simulink model "deadbeat"  (R2018b)
settings: Solver=ode1  StartTime=0.0  StopTime=1  FixedStep=1e-6  RelTol=1e-4
undefined symbols (not defined in the file): Ba, DiscIntNeverNeededParam, flux, Ki, Kp, Ld, Lq, R, Ts
libraries: powerlib x4, simulink x1
settings Model: SimulationMode=accelerator  ExtModeTrigMode=oneshot  ExtModeArmWhenConnect=off  ExtModeAutoUpdateStatusClock=off  Creator=Administrador  LastModifiedBy=123
settings DataIOCC: SaveFormat=Array  SignalLoggingSaveFormat=ModelDataLogs  SignalLoggingName=sigsOut
settings OptimizationCC: BlockReduction=off  BooleanDataType=off  ExpressionDepthLimit=2147483647  InitFltsAndDblsToZero=on  LifeSpan=inf
settings DebuggingCC: SaveWithParameterizedLinksMsg=none  UnderspecifiedInitializationDetection=Classic  MergeDetectMultiDrivingBlocksExec=none  SignalResolutionControl=TryResolveAllWithWarning  MultiTaskDSMMsg=warning  MultiTaskCondExecSysMsg=none  FcnCallInpInsideContextMsg=warning  StateNameClashWarn=warning  LibraryContextMissingDiagnostic=none  SFUnexpectedBacktrackingDiag=warning  SFNoUnconditionalDefaultTransitionDiag=warning  SFExecutionAtInitializationDiag=none
settings HardwareCC: ProdBitPerPointer=32  ProdBitPerSizeT=32  ProdBitPerPtrDiffT=32  ProdLargestAtomicFloat=None  ProdIntDivRoundTo=Undefined  ProdEndianess=Unspecified  ProdWordSize=32  ProdHWDeviceType=32-bit Generic  TargetUnknown=on
settings ModelReferenceCC: PropagateSignalLabelsOutOfModel=off
settings SFSimCC: SimUseLocalCustomCode=off
settings RTWCC: RTWUseLocalCustomCode=off
settings CodeAppCC: StateflowObjectComments=on
settings GRTTargetCC: TargetFcnLib=ansi_tfl_tmw.mat  TargetLangStandard=C89/C90 (ANSI)  GeneratePreprocessorConditionals=Disable all  CombineOutputUpdateFcns=off  GRTInterface=on
settings ConfigComp: CovMetricSettings=dw  CovHtmlReporting=on  CovSaveCumulativeToWorkspaceVar=on  CovSaveSingleToWorkspaceVar=on  CovExternalEMLEnable=off  CovSFcnEnable=off

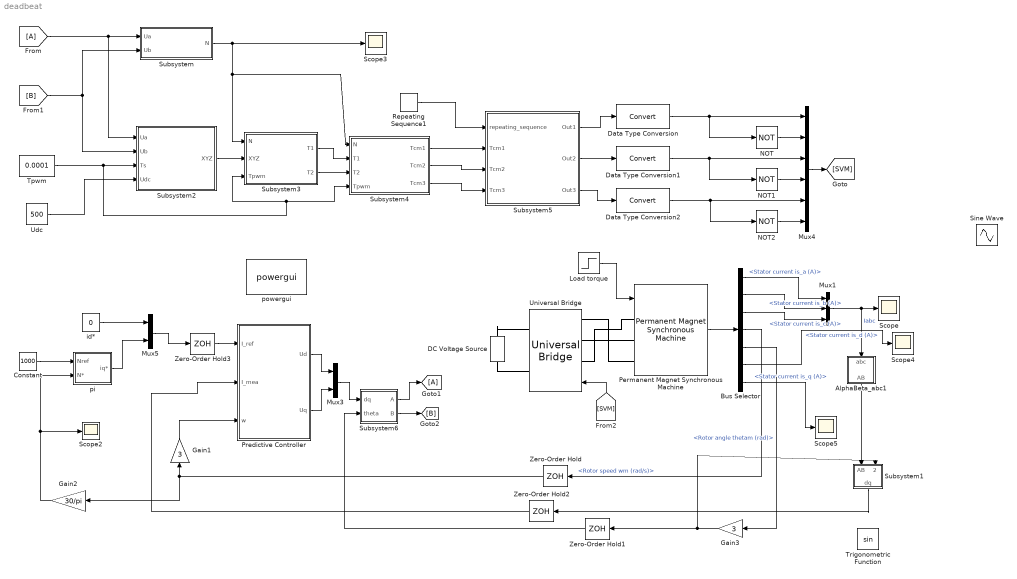
== system deadbeat ==
  AlphaBeta_abc1 : Subsystem
  Bus Selector : BusSelector  OutputSignals=Stator current is_a (A),Stator current is_b (A),Stator current is_c (A),Rotor speed wm (rad/s),Rotor angle thetam (rad),Stator current is_d (A),Stator current is_q (A)
  Constant : Constant  Value=1000
  DC Voltage Source : powerlib/Electrical Sources/DC Voltage Source  Amplitude=500  Measurements=None
      settings: SourceProductName=Simscape Electrical
  Data Type Conversion : DataTypeConversion
  Data Type Conversion1 : DataTypeConversion
  Data Type Conversion2 : DataTypeConversion
  Gain1 : Gain  Gain=3
  Gain2 : Gain  Gain=30/pi
  Gain3 : Gain  Gain=3
  Load torque : Step  Time=0.35  After=5  SampleTime=5e-6
  Mux1 : Mux  Inputs=3
  Mux3 : Mux  Inputs=2
  Mux4 : Mux  Inputs=6
  Mux5 : Mux  Inputs=2
  NOT : Logic  Operator=NOT  IconShape=distinctive  AllPortsSameDT=off  OutDataTypeStr=boolean
  NOT1 : Logic  Operator=NOT  IconShape=distinctive  AllPortsSameDT=off  OutDataTypeStr=boolean
  NOT2 : Logic  Operator=NOT  IconShape=distinctive  AllPortsSameDT=off  OutDataTypeStr=boolean
  Permanent Magnet Synchronous Machine : powerlib/Machines/Permanent Magnet Synchronous Machine  NbPhases=3  FluxDistribution=Sinusoidal  RotorType=Salient-pole  MechanicalLoad=Torque Tm  PresetModel=No  ShowDetailedParameters=on  MeasurementBus=off  Resistance=1.4  Inductance=8.5e-3  dqInductances=[4e-3,6e-3]  La=0.006  MachineConstant=Flux linkage established by magnets (V.s)  Flux=0.09356  VoltageCst=50.9097  TorqueCst=0.42102  Flat=120  Mechanical=[0.0004 0.008 3 0]  PolePairs=4  InitialConditions=[0,0, 0,0]  InitialConditions5ph=[0 0 0 0 0 0]  TsPowergui=0  TsBlock=-1  RefAngle=Aligned with phase A axis (original Park)
  Predictive Controller : MATLAB Function  TreatAsAtomicUnit=on  SystemSampleTime=5e-6
  Repeating Sequence1 : simulink/Sources/Repeating Sequence  rep_seq_t=[0 5e-5 1e-4]  rep_seq_y=[0 5e-5 0]
  Scope{,2..5} (5 alike) : Scope
  Sine Wave : Sin  TimeSource=Use external signal  SampleTime=0
  Subsystem : Subsystem
  Subsystem1 : Subsystem
  Subsystem2 : Subsystem
  Subsystem3 : Subsystem
  Subsystem4 : Subsystem
  Subsystem5 : Subsystem
  Subsystem6 : Subsystem
  Tpwm : Constant  Value=0.0001
  Trigonometric Function : Trigonometry
  "Udc " : Constant  Value=500
  Universal Bridge : powerlib/Power Electronics/Universal Bridge  Arms=3  SnubberResistance=1e5  SnubberCapacitance=inf  Device=IGBT / Diodes  Ron=1e-3  Lon=0  ForwardVoltages="[  0  0  ]"  ForwardVoltage=0  GTOparameters=[ 10e-6 , 20e-6 ]  IGBTparameters=[ 1e-6 , 2e-6 ]  Measurements=None  Measurements_2=None  converterType=Rectifier
      settings: SourceProductName=Simscape Electrical
  Zero-Order Hold{,1..3} (4 alike) : ZeroOrderHold  SampleTime=5e-6
  id* : Constant  Value=0
  pi : Subsystem
  powergui : powerlib/powergui  Priority=1  SimulationMode=Discrete  SampleTime=1e-6  frequency=60  Iterations=50  frequencyindice=0  Pbase=100e6  ErrMax=1e-4  UnitsV=kV  UnitsW=MW  buscounter=0  FunctionMessages=off  echomessages=off  EnableUseOfTLC=off  CurrentSourceSwitches=off  DisableSnubberDevices=off  DisableRonSwitches=off  DisableVfSwitches=off  DisplayEquations=off  SolverType=Tustin  Interpol=off  ExternalGateDelay=off  methode=off  Ts=0  x0status=blocks  SPID=off  SwTol=0  HookPort=off  RestoreLinks=warning  ResistiveCurrentMeasurement=off  Frange=[0:2:500]  Ylog=off  Xlog=on  ShowGrid=off  save=off  variable=ZData  structure=ScopeData1  ZoomFFT=off  StartTime=0.05  cycles=1  DisplayStyle=1  fundamental=50  FreqAxis=off  MaxFrequency=2000  frequencyindicesteady=1  RmsSteady=1  display=off
  wires:
  Mux1/1 -> Scope/1, AlphaBeta_abc1/1(abc)  "Iabc"
  Permanent Magnet Synchronous Machine/1 -> Bus Selector/1
  Bus Selector/1 -> Mux1/1  "<Stator current is_a (A)>"
  Bus Selector/2 -> Mux1/2  "<Stator current is_b (A)>"
  Bus Selector/3 -> Mux1/3  "<Stator current is_c (A)>"
  Constant/1 -> pi/1(Nref)
  Gain2/1 -> pi/2(N*), Scope2/1
  Bus Selector/4 -> Zero-Order Hold/1  "<Rotor speed wm (rad/s)>"
  id*/1 -> Mux5/1
  pi/1(iq*) -> Mux5/2
  Mux5/1 -> Zero-Order Hold3/1
  Gain1/1 -> Predictive Controller/3(w)
  Bus Selector/5 -> Gain3/1  "<Rotor angle thetam (rad)>"
  Gain3/1 -> Zero-Order Hold1/1, Subsystem1/2(theta)
  AlphaBeta_abc1/1(AB) -> Subsystem1/1(AB)
  Subsystem1/1(dq) -> Zero-Order Hold2/1
  Subsystem4/1(Tcm1) -> Subsystem5/2(Tcm1)
  Subsystem/1(N) -> Subsystem4/1(N), Subsystem3/1(N), Scope3/1
  Data Type Conversion/1 -> NOT/1, Mux4/1
  Mux4/1 -> [SVM]
  Subsystem3/2("T2 ") -> Subsystem4/3(T2)
  Subsystem4/2(Tcm2) -> Subsystem5/3(Tcm2)
  NOT2/1 -> Mux4/6
  Subsystem5/2(Out2) -> Data Type Conversion1/1
  Data Type Conversion2/1 -> NOT2/1, Mux4/5
  Subsystem5/3(Out3) -> Data Type Conversion2/1
  NOT/1 -> Mux4/2
  Repeating Sequence1/1 -> Subsystem5/1(repeating_sequence)
  Tpwm/1 -> Subsystem4/4(Tpwm), Subsystem3/3(Tpwm), Subsystem2/3(Ts)
  Subsystem2/1(XYZ) -> Subsystem3/2(XYZ)
  "Udc "/1 -> Subsystem2/4(Udc)
  Data Type Conversion1/1 -> NOT1/1, Mux4/3
  Subsystem5/1(Out1) -> Data Type Conversion/1
  [B] -> Subsystem2/2(Ub), Subsystem/2(Ub)
  NOT1/1 -> Mux4/4
  [A] -> Subsystem2/1(Ua), Subsystem/1(Ua)
  Subsystem3/1(T1) -> Subsystem4/2(T1)
  Subsystem4/3(Tcm3) -> Subsystem5/4(Tcm3)
  [SVM] -> Universal Bridge/1
  Predictive Controller/1(Ud) -> Mux3/1
  Predictive Controller/2(Uq) -> Mux3/2
  Mux3/1 -> Subsystem6/1(dq)
  Subsystem6/2(B) -> [B]
  Subsystem6/1(A) -> [A]
  Zero-Order Hold/1 -> Gain2/1, Gain1/1
  Zero-Order Hold1/1 -> Subsystem6/2(theta)
  Zero-Order Hold2/1 -> Predictive Controller/2(I_mea)
  Zero-Order Hold3/1 -> Predictive Controller/1(I_ref)
  Bus Selector/6 -> Scope4/1  "<Stator current is_d (A)>"
  Bus Selector/7 -> Scope5/1  "<Stator current is_q (A)>"
  Load torque/1 -> Permanent Magnet Synchronous Machine/1
  connections:
  DC Voltage Source/RConn1 -- Universal Bridge/RConn1
  DC Voltage Source/LConn1 -- Universal Bridge/RConn2
  Universal Bridge/LConn3 -- Permanent Magnet Synchronous Machine/LConn3
  Permanent Magnet Synchronous Machine/LConn2 -- Universal Bridge/LConn2
  Universal Bridge/LConn1 -- Permanent Magnet Synchronous Machine/LConn1

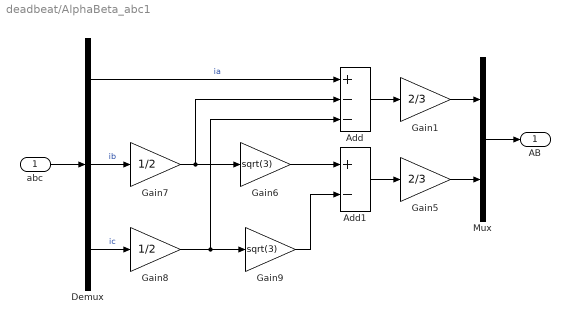
== system deadbeat/AlphaBeta_abc1 ==
  abc : Inport
  Add : Sum  Inputs=+--
  Add1 : Sum  Inputs=+-
  Demux : Demux  Outputs=3
  Gain1 : Gain  Gain=2/3
  Gain5 : Gain  Gain=2/3
  Gain6 : Gain  Gain=sqrt(3)
  Gain7 : Gain  Gain=1/2
  Gain8 : Gain  Gain=1/2
  Gain9 : Gain  Gain=sqrt(3)
  Mux : Mux  Inputs=2
  AB : Outport
  wires:
  abc/1 -> Demux/1
  Demux/2 -> Gain7/1  "ib"
  Demux/3 -> Gain8/1  "ic"
  Add/1 -> Gain1/1
  Gain7/1 -> Gain6/1, Add/2
  Gain8/1 -> Gain9/1, Add/3
  Gain6/1 -> Add1/1
  Gain9/1 -> Add1/2
  Demux/1 -> Add/1  "ia"
  Add1/1 -> Gain5/1
  Gain1/1 -> Mux/1
  Gain5/1 -> Mux/2
  Mux/1 -> AB/1

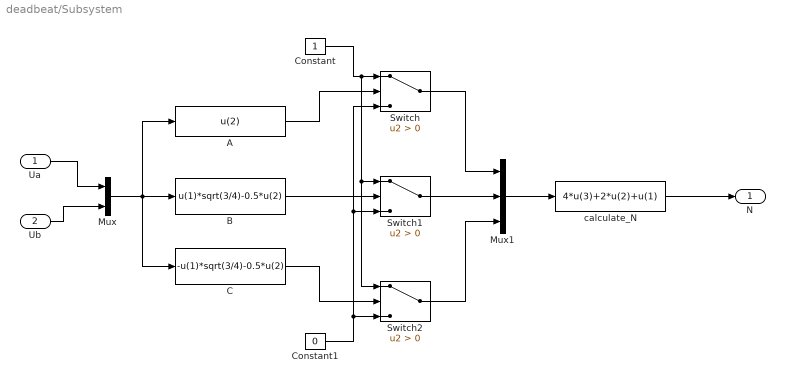
== system deadbeat/Subsystem ==
  Ua : Inport
  Ub : Inport  Port=2
  A : Fcn  Expr=u(2)
  B : Fcn  Expr=u(1)*sqrt(3/4)-0.5*u(2)
  C : Fcn  Expr=-u(1)*sqrt(3/4)-0.5*u(2)
  Constant : Constant
  Constant1 : Constant  Value=0
  Mux : Mux  Inputs=2
  Mux1 : Mux  Inputs=3
  Switch : Switch  Criteria=u2 > Threshold
  Switch1 : Switch  Criteria=u2 > Threshold
  Switch2 : Switch  Criteria=u2 > Threshold
  calculate_N : Fcn  Expr=4*u(3)+2*u(2)+u(1)
  N : Outport
  wires:
  Ua/1 -> Mux/1
  Ub/1 -> Mux/2
  Mux/1 -> A/1, B/1, C/1
  Constant/1 -> Switch2/1, Switch1/1, Switch/1
  Constant1/1 -> Switch2/3, Switch1/3, Switch/3
  A/1 -> Switch/2
  B/1 -> Switch1/2
  C/1 -> Switch2/2
  Switch/1 -> Mux1/1
  Switch1/1 -> Mux1/2
  Switch2/1 -> Mux1/3
  Mux1/1 -> calculate_N/1
  calculate_N/1 -> N/1

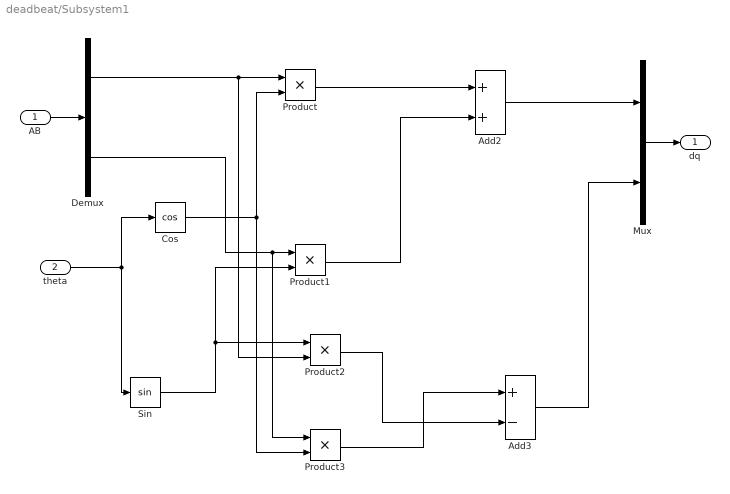
== system deadbeat/Subsystem1 ==
  AB : Inport
  theta : Inport  Port=2
  Add2 : Sum
  Add3 : Sum  Inputs=+-
  Cos : Trigonometry  Operator=cos
  Demux : Demux  Outputs=2
  Mux : Mux  Inputs=2
  Product{,1..3} (4 alike) : Product
  Sin : Trigonometry
  dq : Outport
  wires:
  Product2/1 -> Add3/2
  Product/1 -> Add2/1
  theta/1 -> Sin/1, Cos/1
  Mux/1 -> dq/1
  AB/1 -> Demux/1
  Add3/1 -> Mux/2
  Add2/1 -> Mux/1
  Cos/1 -> Product3/2, Product/2
  Demux/2 -> Product1/1, Product3/1
  Demux/1 -> Product/1, Product2/2
  Product1/1 -> Add2/2
  Product3/1 -> Add3/1
  Sin/1 -> Product2/1, Product1/2

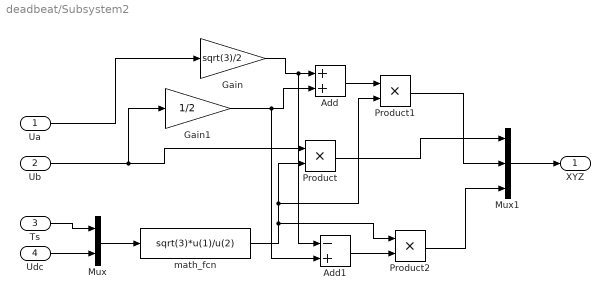
== system deadbeat/Subsystem2 ==
  Ua : Inport
  Ub : Inport  Port=2
  Ts : Inport  Port=3
  Udc : Inport  Port=4
  Add : Sum
  Add1 : Sum  Inputs=-+
  Gain : Gain  Gain=sqrt(3)/2
  Gain1 : Gain  Gain=1/2
  Mux : Mux  Inputs=2
  Mux1 : Mux  Inputs=3
  Product : Product
  Product1 : Product
  Product2 : Product
  math_fcn : Fcn  Expr=sqrt(3)*u(1)/u(2)
  XYZ : Outport
  wires:
  Mux/1 -> math_fcn/1
  Ts/1 -> Mux/1
  Udc/1 -> Mux/2
  Mux1/1 -> XYZ/1
  math_fcn/1 -> Product2/1, Product1/2, Product/2
  Product/1 -> Mux1/1
  Ua/1 -> Gain/1
  Gain/1 -> Add1/1, Add/1
  Ub/1 -> Gain1/1, Product/1
  Add/1 -> Product1/1
  Product1/1 -> Mux1/2
  Add1/1 -> Product2/2
  Product2/1 -> Mux1/3
  Gain1/1 -> Add1/2, Add/2

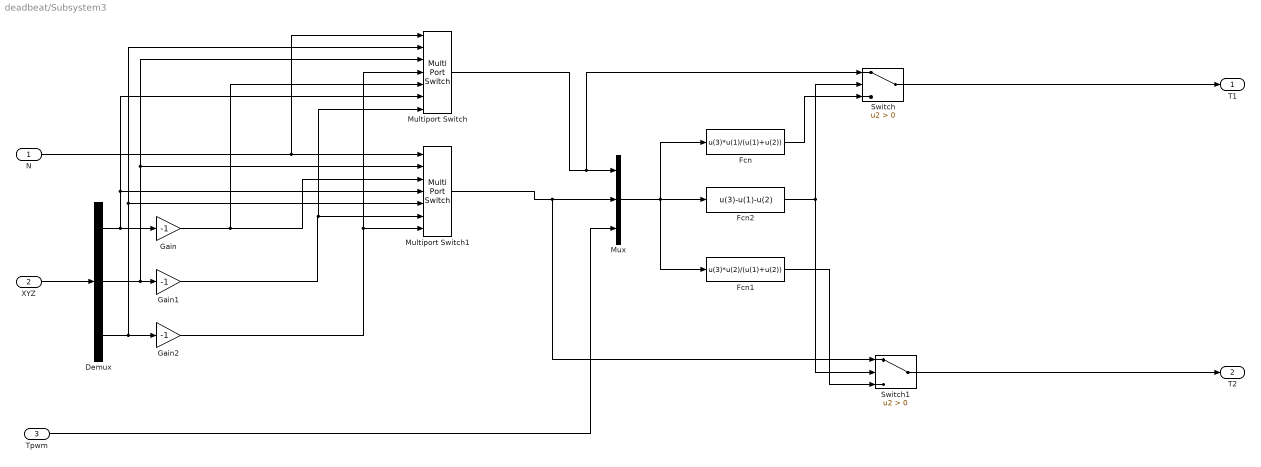
== system deadbeat/Subsystem3 ==
  N : Inport
  XYZ : Inport  Port=2
  Tpwm : Inport  Port=3
  Demux : Demux  Outputs=3
  Fcn : Fcn  Expr=u(3)*u(1)/(u(1)+u(2))
  Fcn1 : Fcn  Expr=u(3)*u(2)/(u(1)+u(2))
  Fcn2 : Fcn  Expr=u(3)-u(1)-u(2)
  Gain : Gain  Gain=-1
  Gain1 : Gain  Gain=-1
  Gain2 : Gain  Gain=-1
  Multiport Switch : MultiPortSwitch  Inputs=6
  Multiport Switch1 : MultiPortSwitch  Inputs=6
  Mux : Mux  Inputs=3
  Switch : Switch  Criteria=u2 > Threshold
  Switch1 : Switch  Criteria=u2 > Threshold
  T1 : Outport
  "T2 " : Outport  Port=2
  wires:
  XYZ/1 -> Demux/1
  N/1 -> Multiport Switch/1, Multiport Switch1/1
  Demux/1 -> Multiport Switch/6, Multiport Switch1/4, Gain/1
  Demux/2 -> Multiport Switch1/2, Multiport Switch/3, Gain1/1
  Demux/3 -> Multiport Switch1/5, Multiport Switch/2, Gain2/1
  Gain/1 -> Multiport Switch/5, Multiport Switch1/3
  Gain2/1 -> Multiport Switch1/7, Multiport Switch/4
  Gain1/1 -> Multiport Switch/7, Multiport Switch1/6
  Multiport Switch/1 -> Switch/1, Mux/1
  Multiport Switch1/1 -> Switch1/1, Mux/2
  Tpwm/1 -> Mux/3
  Switch1/1 -> "T2 "/1
  Switch/1 -> T1/1
  Fcn2/1 -> Switch/2, Switch1/2
  Mux/1 -> Fcn1/1, Fcn/1, Fcn2/1
  Fcn/1 -> Switch/3
  Fcn1/1 -> Switch1/3

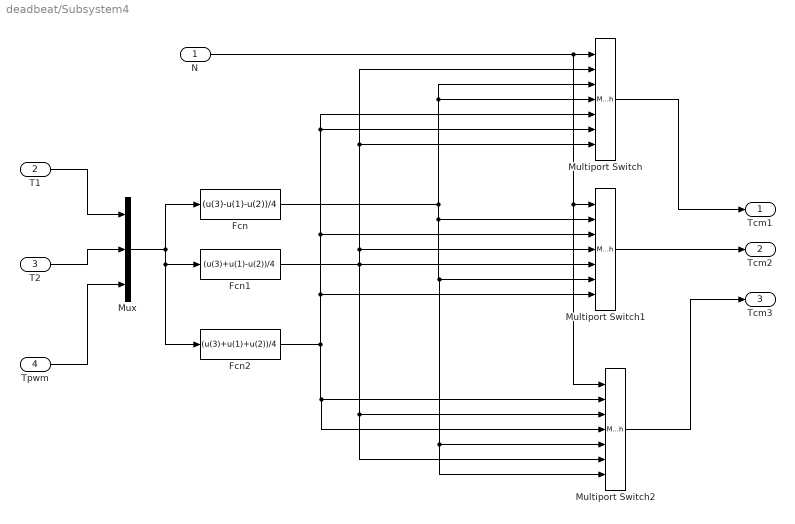
== system deadbeat/Subsystem4 ==
  N : Inport
  T1 : Inport  Port=2
  T2 : Inport  Port=3
  Tpwm : Inport  Port=4
  Fcn : Fcn  Expr=(u(3)-u(1)-u(2))/4
  Fcn1 : Fcn  Expr=(u(3)+u(1)-u(2))/4
  Fcn2 : Fcn  Expr=(u(3)+u(1)+u(2))/4
  Multiport Switch : MultiPortSwitch  Inputs=6
  Multiport Switch1 : MultiPortSwitch  Inputs=6
  Multiport Switch2 : MultiPortSwitch  Inputs=6
  Mux : Mux  Inputs=3
  Tcm1 : Outport
  Tcm2 : Outport  Port=2
  Tcm3 : Outport  Port=3
  wires:
  N/1 -> Multiport Switch2/1, Multiport Switch1/1, Multiport Switch/1
  T1/1 -> Mux/1
  T2/1 -> Mux/2
  Tpwm/1 -> Mux/3
  Mux/1 -> Fcn2/1, Fcn1/1, Fcn/1
  Fcn/1 -> Multiport Switch2/7, Multiport Switch2/5, Multiport Switch1/6, Multiport Switch1/2, Multiport Switch/4, Multiport Switch/3
  Fcn1/1 -> Multiport Switch2/6, Multiport Switch2/3, Multiport Switch1/5, Multiport Switch1/4, Multiport Switch/7, Multiport Switch/2
  Fcn2/1 -> Multiport Switch2/4, Multiport Switch2/2, Multiport Switch1/7, Multiport Switch1/3, Multiport Switch/6, Multiport Switch/5
  Multiport Switch/1 -> Tcm1/1
  Multiport Switch1/1 -> Tcm2/1
  Multiport Switch2/1 -> Tcm3/1

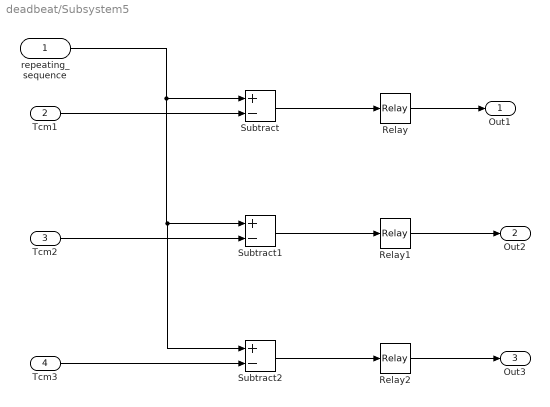
== system deadbeat/Subsystem5 ==
  repeating_sequence : Inport
  Tcm1 : Inport  Port=2
  Tcm2 : Inport  Port=3
  Tcm3 : Inport  Port=4
  Relay : Relay
  Relay1 : Relay
  Relay2 : Relay
  Subtract : Sum  Inputs=+-
  Subtract1 : Sum  Inputs=+-
  Subtract2 : Sum  Inputs=+-
  Out1 : Outport
  Out2 : Outport  Port=2
  Out3 : Outport  Port=3
  wires:
  repeating_sequence/1 -> Subtract2/1, Subtract1/1, Subtract/1
  Tcm1/1 -> Subtract/2
  Tcm2/1 -> Subtract1/2
  Tcm3/1 -> Subtract2/2
  Subtract/1 -> Relay/1
  Subtract1/1 -> Relay1/1
  Subtract2/1 -> Relay2/1
  Relay1/1 -> Out2/1
  Relay/1 -> Out1/1
  Relay2/1 -> Out3/1

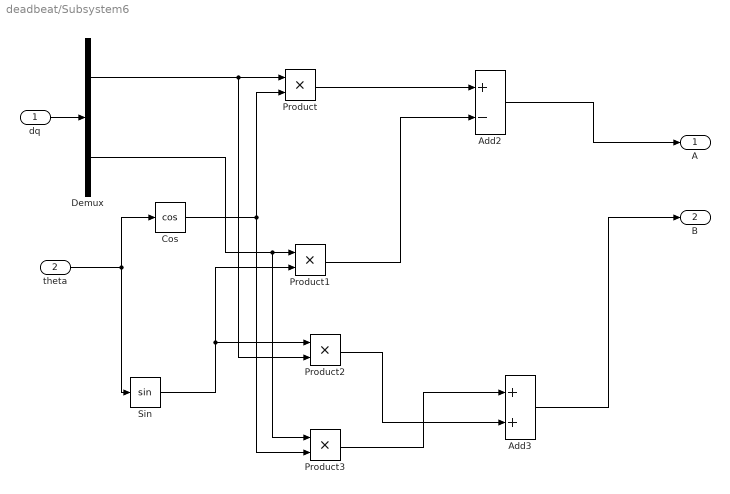
== system deadbeat/Subsystem6 ==
  dq : Inport
  theta : Inport  Port=2
  Add2 : Sum  Inputs=+-
  Add3 : Sum
  Cos : Trigonometry  Operator=cos
  Demux : Demux  Outputs=2
  Product{,1..3} (4 alike) : Product
  Sin : Trigonometry
  A : Outport
  B : Outport  Port=2
  wires:
  Sin/1 -> Product1/2, Product2/1
  Product3/1 -> Add3/1
  Product1/1 -> Add2/2
  Demux/1 -> Product2/2, Product/1
  Demux/2 -> Product3/1, Product1/1
  Cos/1 -> Product/2, Product3/2
  Add3/1 -> B/1
  dq/1 -> Demux/1
  Add2/1 -> A/1
  theta/1 -> Cos/1, Sin/1
  Product/1 -> Add2/1
  Product2/1 -> Add3/2

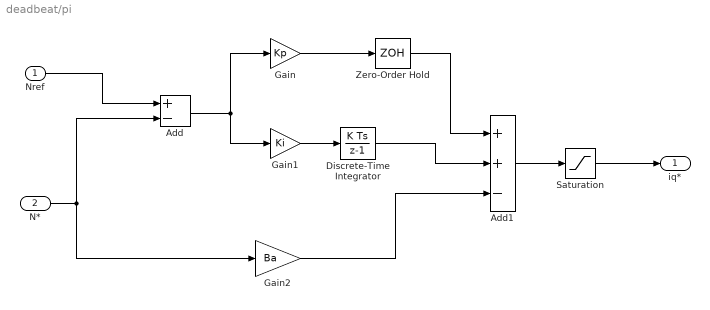
== system deadbeat/pi ==
  Nref : Inport
  N* : Inport  Port=2
  Add : Sum  Inputs=+-
  Add1 : Sum  Inputs=++-
  Discrete-Time Integrator : DiscreteIntegrator  SampleTime=-1  ICPrevOutput=DiscIntNeverNeededParam  ICPrevScaledInput=DiscIntNeverNeededParam
  Gain : Gain  Gain=Kp
  Gain1 : Gain  Gain=Ki
  Gain2 : Gain  Gain=Ba
  Saturation : Saturate  UpperLimit=18  LowerLimit=-18
  Zero-Order Hold : ZeroOrderHold  SampleTime=-1
  iq* : Outport
  wires:
  Nref/1 -> Add/1
  N*/1 -> Gain2/1, Add/2
  Add/1 -> Gain1/1, Gain/1
  Gain/1 -> Zero-Order Hold/1
  Zero-Order Hold/1 -> Add1/1
  Gain1/1 -> Discrete-Time Integrator/1
  Discrete-Time Integrator/1 -> Add1/2
  Gain2/1 -> Add1/3
  Add1/1 -> Saturation/1
  Saturation/1 -> iq*/1

== matlab function deadbeat/Predictive Controller ==
  settings: updateMethod=DISCRETE  sampleTime=Ts
  data: I_ref input; I_mea input; Ts parameter; w input; R parameter; Ld parameter; Ud output; Uq output; flux parameter; Lq parameter

function [Ud,Uq] = control(I_ref,I_mea,Ts,w,R,Ld,flux, Lq)
id = I_mea(1);
iq = I_mea(2);
idr = I_ref(1);
iqr = I_ref(2);
Ud = R*id + Ld*(idr-id)/Ts - w*Ld*iq;
Uq = R*iq + Lq*(iqr-iq)/Ts + w*Lq*id + w*flux;
end
